simulink model "car5"  (R2016a)
settings: Solver=VariableStepAuto  StartTime=0.0  StopTime=20  RelTol=1e-3
values from neighbouring files (symbols this model uses):
  LK1 = -LK1    [car.m]    (also in car_m.m = [-1 0;0 -1]')
  x0 = [1 3 2 1 3 2 4 5]'    [car.m]    (also in car_m.m = [0 0]')
libraries: simulink x1
settings Model: Creator=richa  LastModifiedBy=108

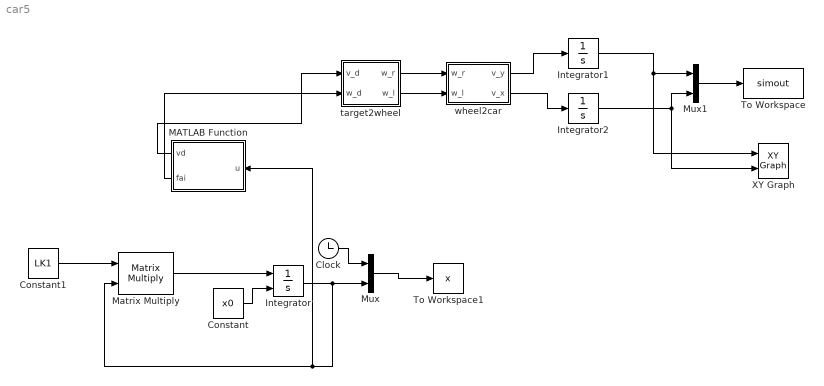
== system car5 ==
  Clock : Clock
  Constant : Constant  Value=x0
  Constant1 : Constant  Value=LK1  VectorParams1D=off
  Integrator : Integrator  InitialConditionSource=external
  Integrator1 : Integrator
  Integrator2 : Integrator
  MATLAB Function : MATLAB Function  TreatAsAtomicUnit=on
  Matrix Multiply : Product  Multiplication=Matrix(*)
  Mux : Mux  Inputs=2
  Mux1 : Mux  Inputs=2
  To Workspace : ToWorkspace  VariableName=simout  SampleTime=-1
  To Workspace1 : ToWorkspace  VariableName=x  SampleTime=-1
  XY Graph : simulink/Sinks/XY Graph  xmin=-2  xmax=2  ymin=-2  ymax=2  st=0
  target2wheel : Subsystem
  wheel2car : Subsystem
  wires:
  Integrator1/1 -> Mux1/1, XY Graph/1
  Integrator2/1 -> Mux1/2, XY Graph/2
  Mux1/1 -> To Workspace/1
  wheel2car/1(v_y) -> Integrator1/1
  wheel2car/2(v_x) -> Integrator2/1
  target2wheel/1(w_r) -> wheel2car/1(w_r)
  target2wheel/2(w_l) -> wheel2car/2(w_l)
  Constant/1 -> Integrator/2
  Mux/1 -> To Workspace1/1
  Clock/1 -> Mux/1
  Matrix Multiply/1 -> Integrator/1
  Constant1/1 -> Matrix Multiply/1
  Integrator/1 -> Mux/2, MATLAB Function/1(u), Matrix Multiply/2
  MATLAB Function/1(vd) -> target2wheel/1(v_d)
  MATLAB Function/2(fai) -> target2wheel/2(w_d)

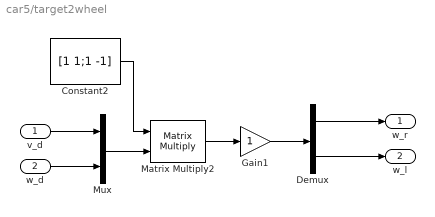
== system car5/target2wheel ==
  v_d : Inport
  w_d : Inport  Port=2
  Constant2 : Constant  Value=[1 1;1 -1]
  Demux : Demux  Outputs=2
  Gain1 : Gain
  Matrix Multiply2 : Product  Multiplication=Matrix(*)
  Mux : Mux  Inputs=2
  w_r : Outport
  w_l : Outport  Port=2
  wires:
  Mux/1 -> Matrix Multiply2/2
  Gain1/1 -> Demux/1
  Constant2/1 -> Matrix Multiply2/1
  Matrix Multiply2/1 -> Gain1/1
  v_d/1 -> Mux/1
  w_d/1 -> Mux/2
  Demux/2 -> w_l/1
  Demux/1 -> w_r/1

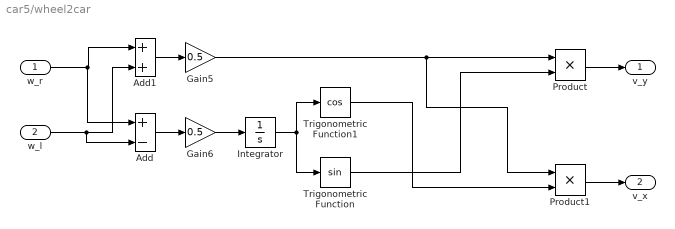
== system car5/wheel2car ==
  w_r : Inport
  w_l : Inport  Port=2
  Add : Sum  Inputs=+-
  Add1 : Sum
  Gain5 : Gain  Gain=0.5
  Gain6 : Gain  Gain=0.5
  Integrator : Integrator
  Product : Product
  Product1 : Product
  Trigonometric Function : Trigonometry
  Trigonometric Function1 : Trigonometry  Operator=cos
  v_y : Outport
  v_x : Outport  Port=2
  wires:
  Gain5/1 -> Product1/1, Product/1
  Gain6/1 -> Integrator/1
  Integrator/1 -> Trigonometric Function1/1, Trigonometric Function/1
  Trigonometric Function/1 -> Product/2
  Trigonometric Function1/1 -> Product1/2
  Product/1 -> v_y/1
  w_r/1 -> Add/1, Add1/1
  w_l/1 -> Add/2, Add1/2
  Product1/1 -> v_x/1
  Add1/1 -> Gain5/1
  Add/1 -> Gain6/1

== matlab function car5/MATLAB Function ==
  data: u input; vd output; fai output
function [vd,fai]  = fcn(u)
%#codegen

vd=[0];
fai=[0];
j=1;
for i=1:1
   vd(j) = sqrt(u(i).^2+ u(i+1).^2);
   fai(j) = atan(u(i+1)/u(i));
   j=j+1;
end

end
